simulink model "lazo_cerrado"  (R2021b)
settings: Solver=VariableStepAuto  StartTime=0.0  StopTime=25  RelTol=1e-3
settings Model: Creator=axel_  LastModifiedBy=axel_

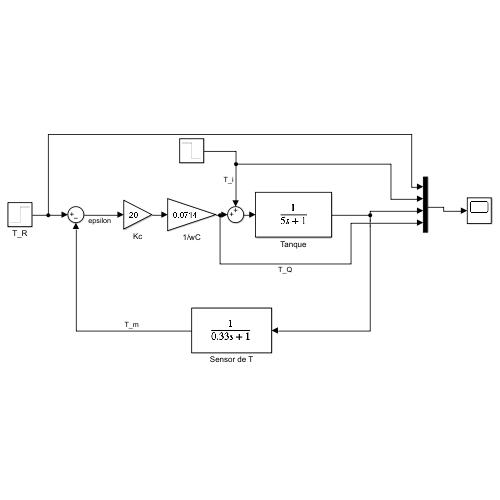
[thumbnail: Simulink's stored preview of the top-level diagram]
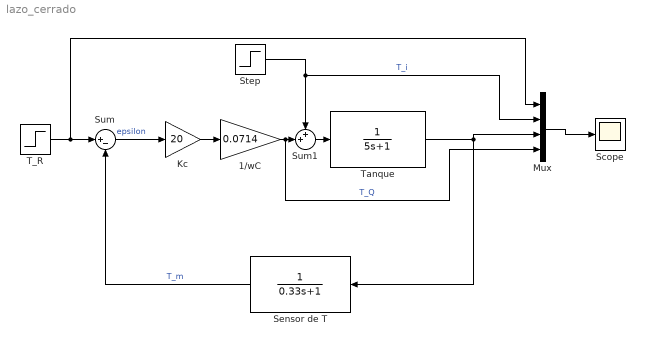
== system lazo_cerrado ==
  1/wC : Gain  Gain=0.0714
  Kc : Gain  Gain=20
  Mux : Mux
  Scope : Scope
  Sensor de T : TransferFcn  Denominator=[0.33 1]
  Step : Step  After=-5  SampleTime=0
  Sum : Sum  Inputs=|+-
  Sum1 : Sum  Inputs=++|
  T_R : Step  After=0  SampleTime=0
  Tanque : TransferFcn  Denominator=[5 1]
  wires:
  Mux/1 -> Scope/1
  Tanque/1 -> Sensor de T/1, Mux/3
  Sensor de T/1 -> Sum/2  "T_m"
  T_R/1 -> Mux/1, Sum/1
  Sum/1 -> Kc/1  "epsilon"
  Kc/1 -> 1/wC/1
  1/wC/1 -> Mux/4, Sum1/2  "T_Q"
  Sum1/1 -> Tanque/1
  Step/1 -> Mux/2, Sum1/1  "T_i"
